simulink model "Simulatore_digitale_5"  (Simulink 7.7)
settings: Solver=ode3  StartTime=0.0  StopTime=2*stop_t  FixedStep=Ts  MaxStep=Ts/10  MinStep=Ts/100  RelTol=1e-3
values from neighbouring files (symbols this model uses):
  a_da = 0    [CA_GIUSE.m]    (also in Script.m)
  a_dp = 2e-2    (= 0.02)    [CA_GIUSE.m]    (also in Script.m = 0)
  a_ds = 0e-1    (= 0)    [CA_GIUSE.m]    (also in Script.m)
  aph = 0.05    [CA_GIUSE.m]    (also in Script.m)
  Da_c = 0e-3    (= 0)    [CA_GIUSE.m]    (also in Script.m)
  Da_r = 00e-1    (= 0)    [CA_GIUSE.m]    (also in Script.m)
  Dp_c = 00e-3    (= 0)    [CA_GIUSE.m]    (also in Script.m)
  Dp_r = 00e-1    (= 0)    [CA_GIUSE.m]    (also in Script.m)
  Ds_c = 00e-3    (= 0)    [CA_GIUSE.m]    (also in Script.m)
  Ds_r = 00e-1    (= 0)    [CA_GIUSE.m]    (also in Script.m)
  e_ds = 0e-4    (= 0)    [CA_GIUSE.m]    (also in Script.m)
  e_r = 0e-1    (= 0)    [CA_GIUSE.m]    (also in Script.m)
  Ga = 0e-3    (= 0)    [CA_GIUSE.m]    (also in Script.m)
  Gda = 0    [CA_GIUSE.m]    (also in Script.m = 1)
  Gdp = 0    [CA_GIUSE.m]    (also in Script.m = 1)
  Gf = 1/(Kd*Gs)    [CA_GIUSE.m]    (also in Script.m)
  Gr = 0e0    (= 0)    [CA_GIUSE.m]    (also in Script.m = 1)
  Gs = 0e-0    (= 0)    [CA_GIUSE.m]    (also in Script.m)
  Kd = 0    [CA_GIUSE.m]    (also in Script.m)
  lp_bssl_d = 1    [CA_GIUSE.m]    (also in Script.m)
  lp_bssl_n = 1    [CA_GIUSE.m]    (also in Script.m)
  over = 0.1    [CA_GIUSE.m]    (also in Script.m = 0)
  Pulse_da = 0    [CA_GIUSE.m]    (also in Script.m)
  Pulse_dp = 0e-3    (= 0)    [CA_GIUSE.m]    (also in Script.m)
  Pulse_ds = 0    [CA_GIUSE.m]    (also in Script.m)
  R_0 = 1    [CA_GIUSE.m]    (also in Script.m)
  sig_gen_amp = 1    [CA_GIUSE.m]    (also in Script.m = 0.5)
  sig_gen_freq = 0.5    [CA_GIUSE.m]    (also in Script.m = 0.25)
  Ts = 0.1/(Wceff); [Gcz,Lz]=TDmode(Ts,Glp,Gc,Ga,Gp,Gs,Gf)    [CA_GIUSE.m]    (also in Script.m)
undefined symbols (not defined in the file or in its folder): den_Gcz, den_Gda, den_Gdp, den_Gp, num_Gcz, num_Gda, num_Gdp, num_Gp
libraries: simulink x14
settings Model: Creator=Sandro  LastModifiedBy=giuse

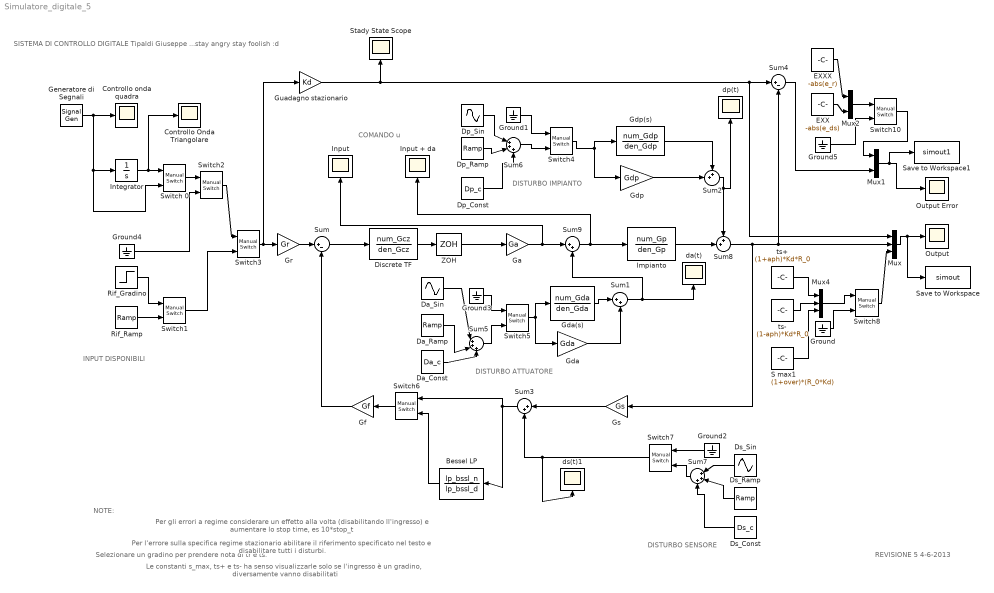
== system Simulatore_digitale_5 ==
  note: SISTEMA DI CONTROLLO  DIGITALE
      | Tipaldi Giuseppe
      |
      | ...stay angry stay foolish
      | :d
  note: DISTURBO ATTUATORE
  note: DISTURBO IMPIANTO
  note: INPUT DISPONIBILI
  note: COMANDO u
  note: DISTURBO SENSORE
  note: NOTE:
  note: Per gli errori a regime considerare un effetto alla volta (disabilitando ll'ingresso) e aumentare lo stop time, es 10*stop_t
  note: Selezionare un gradino per prendere nota di tr e ts.
  note: Per l'errore sulla specifica regime stazionario abilitare il riferimento specificato nel testo e disabilitare tutti i disturbi.
  note: Le constanti s_max, ts+ e ts- ha senso visualizzarle solo se l'ingresso è un gradino, diversamente vanno disabilitati
  note: REVISIONE 5
      | 4-6-2013
  " Switch 0" : simulink/Signal Routing/Manual Switch  SystemSampleTime=-1  sw=1  action=0  varsize=off
   Switch{1..2,4..5,7..8,10} (7 alike) : simulink/Signal Routing/Manual Switch  SystemSampleTime=-1  sw=1  action=0  varsize=off
  " Switch3" : simulink/Signal Routing/Manual Switch  SystemSampleTime=-1  sw=0  action=0  varsize=off
  " Switch6" : simulink/Signal Routing/Manual Switch  SystemSampleTime=-1  sw=0  action=0  varsize=off
  Bessel LP : TransferFcn  Numerator=lp_bssl_n  Denominator=lp_bssl_d
  Controllo Onda Triangolare : Scope
      settings: SaveName=ScopeData3
  Controllo onda quadra : Scope
      settings: TimeRange=0.002216033935546875  YMin=2.1909418072197  YMax=2.191153294711311  SaveName=ScopeData6
  Da_Const : Constant  Value=Da_c
  Da_Ramp : simulink/Sources/Ramp  SystemSampleTime=-1  slope=Da_r  start=0  X0=0
  Da_Sin : Sin  Amplitude=a_da  Frequency=Pulse_da  SampleTime=0
  Discrete TF : DiscreteTransferFcn  Numerator=num_Gcz  Denominator=den_Gcz  SampleTime=Ts
  Dp_Const : Constant  Value=Dp_c
  Dp_Ramp : simulink/Sources/Ramp  SystemSampleTime=-1  slope=Dp_r  start=0  X0=0
  Dp_Sin : Sin  Amplitude=a_dp  Frequency=Pulse_dp  SampleTime=0
  Ds_Const : Constant  Value=Ds_c
  Ds_Ramp : simulink/Sources/Ramp  SystemSampleTime=-1  slope=Ds_r  start=0  X0=0
  Ds_Sin : Sin  Amplitude=a_ds  Frequency=Pulse_ds  SampleTime=0
  EXX : Constant  Value=-abs(e_ds)
  EXXX : Constant  Value=-abs(e_r)
  Ga : Gain  Gain=Ga
  Gda : Gain  Gain=Gda
  Gda(s) : TransferFcn  Numerator=num_Gda  Denominator=den_Gda
  Gdp : Gain  Gain=Gdp
  Gdp(s) : TransferFcn  Numerator=num_Gdp  Denominator=den_Gdp
  Generatore di Segnali : SignalGenerator  WaveForm=square  Amplitude=sig_gen_amp  Frequency=sig_gen_freq  Units=rad/sec
  Gf : Gain  Gain=Gf
  Gr : Gain  Gain=Gr
  Ground{,1..5} (6 alike) : Ground
  Gs : Gain  Gain=Gs
  Guadagno stazionario : Gain  Gain=Kd
  Impianto : TransferFcn  Numerator=num_Gp  Denominator=den_Gp
  Input : Scope
      settings: TimeRange=7.62942779291553  YMin=0.9536585365853658  YMax=1.036585365853659  SaveName=ScopeData4
  Input + da : Scope
      settings: TimeRange=7.62942779291553  YMin=0.9536585365853658  YMax=1.036585365853659
  Integrator : Integrator  InitialCondition=0.5
  Mux : Mux  Inputs=3
  Mux1 : Mux  Inputs=2
  Mux2 : Mux  Inputs=2
  Mux4 : Mux  Inputs=3
  "Output " : Scope
      settings: TimeRange=1.6  YMin=-3.580716253443526e+244  YMax=-3.80716253443527e+243
  Output Error : Scope
      settings: TimeRange=2  YMin=-0.003785942087987625  YMax=-0.003563613211040456  SaveName=ScopeData2
  Rif_Gradino : Step  Time=0  After=R_0  SampleTime=0
  Rif_Ramp : simulink/Sources/Ramp  SystemSampleTime=-1  slope=R_0  start=0  X0=0
  S max1 : Constant  Value=(1+over)*(R_0*Kd)
  Save to Workspace : ToWorkspace  VariableName=simout  SampleTime=-1  SaveFormat=Structure With Time
  Save to Workspace1 : ToWorkspace  VariableName=simout1  SampleTime=-1  SaveFormat=Structure With Time
  Stady State Scope : Scope
      settings: TimeRange=7.62942779291553  YMin=0.9536585365853658  YMax=1.036585365853659  SaveName=ScopeData7
  Sum : Sum  Inputs=|+-
  Sum1 : Sum  Inputs=|++
  Sum2 : Sum  Inputs=++|
  Sum3 : Sum  Inputs=|++
  Sum4 : Sum  Inputs=|+-
  Sum5 : Sum  Inputs=|+++
  Sum6 : Sum  Inputs=|+++
  Sum7 : Sum  Inputs=|+++
  Sum8 : Sum  Inputs=++|
  Sum9 : Sum  Inputs=|++
  ZOH : ZeroOrderHold  SampleTime=Ts
  da(t) : Scope
      settings: TimeRange=7.62942779291553  YMin=0.9536585365853658  YMax=1.036585365853659  SaveName=ScopeData8
  dp(t) : Scope
      settings: TimeRange=7.62942779291553  YMin=0.9536585365853658  YMax=1.036585365853659  SaveName=ScopeData5
  ds(t)1 : Scope
      settings: TimeRange=7.62942779291553  YMin=0.9536585365853658  YMax=1.036585365853659  SaveName=ScopeData9
  ts+ : Constant  Value=(1+aph)*Kd*R_0
  ts- : Constant  Value=(1-aph)*Kd*R_0
  wires:
  Sum9/1 -> Impianto/1, Input + da/1
  Guadagno stazionario/1 -> Sum4/1, Mux/1, Stady State Scope/1
  Mux/1 -> "Output "/1, Save to Workspace/1
  Gs/1 -> Sum3/1
  Rif_Ramp/1 -> " Switch1"/2
  Rif_Gradino/1 -> " Switch1"/1
  ts+/1 -> Mux4/1
  Mux4/1 -> " Switch8"/1
  Ground/1 -> " Switch8"/2
  Generatore di Segnali/1 -> Controllo onda quadra/1, Integrator/1, " Switch 0"/2
  Sum3/1 -> Bessel LP/1, " Switch6"/1
  Gf/1 -> Sum/2
  " Switch6"/1 -> Gf/1
  Bessel LP/1 -> " Switch6"/2
  Ga/1 -> Input/1, Sum9/1
  " Switch 0"/1 -> " Switch2"/1
  Ground4/1 -> " Switch2"/2
  Integrator/1 -> Controllo Onda Triangolare/1, " Switch 0"/1
  " Switch8"/1 -> Mux/3
  Gdp(s)/1 -> Sum2/1
  ts-/1 -> Mux4/2
  S max1/1 -> Mux4/3
  Sum5/1 -> " Switch5"/2
  Ground3/1 -> " Switch5"/1
  " Switch5"/1 -> Gda(s)/1, Gda/1
  " Switch4"/1 -> Gdp(s)/1, Gdp/1
  Ground2/1 -> " Switch7"/1
  " Switch7"/1 -> Sum3/2, ds(t)1/1
  Da_Const/1 -> Sum5/3
  Da_Ramp/1 -> Sum5/2
  Da_Sin/1 -> Sum5/1
  Dp_Const/1 -> Sum6/3
  Dp_Ramp/1 -> Sum6/2
  Dp_Sin/1 -> Sum6/1
  Sum7/1 -> " Switch7"/2
  Ds_Sin/1 -> Sum7/1
  Ds_Ramp/1 -> Sum7/2
  Ds_Const/1 -> Sum7/3
  Sum6/1 -> " Switch4"/2
  Gr/1 -> Sum/1
  Gdp/1 -> Sum2/2
  Sum2/1 -> Sum8/1, dp(t)/1
  Impianto/1 -> Sum8/2
  Sum8/1 -> Gs/1, Mux/2, Sum4/2
  Gda(s)/1 -> Sum1/1
  Gda/1 -> Sum1/2
  Sum1/1 -> Sum9/2, da(t)/1
  Mux1/1 -> Output Error/1, Save to Workspace1/1
  Sum4/1 -> Mux1/2
  Discrete TF/1 -> ZOH/1
  ZOH/1 -> Ga/1
  Sum/1 -> Discrete TF/1
  " Switch2"/1 -> " Switch3"/1
  " Switch1"/1 -> " Switch3"/2
  Ground1/1 -> " Switch4"/1
  " Switch3"/1 -> Gr/1, Guadagno stazionario/1
  EXXX/1 -> Mux2/1
  EXX/1 -> Mux2/2
  Ground5/1 -> " Switch10"/2
  Mux2/1 -> " Switch10"/1
  " Switch10"/1 -> Mux1/1
